simulink model "nfo"  (R2023b)
settings: Solver=FixedStepAuto  StartTime=0.0  StopTime=10.0  FixedStep=1e-4  RelTol=1e-3
values from neighbouring files (symbols this model uses):
  flux = 0.0059    [nfo.sldd]
  if_init = 40.0    [nfo.sldd]
  L = 8.5E-5    [nfo.sldd]
  Pn = 5.0    [nfo.sldd]
  Rs = 0.035    [nfo.sldd]
  Ts = 0.0001    [nfo.sldd]
  Udc = 24.0    [nfo.sldd]
undefined symbols (not defined in the file or in its folder): DiscIntNeverNeededParam, magnitude, PLL_I, PLL_P, sigbuilder_block
libraries: slpidlib x4, dspstat3 x1, mcbplantlib x1, autolibpmsmexterior x1
(part 2 of 2)

== matlab function nfo/Algorithm/Enabled Subsystem/MATLAB Function ==
  data: Time input; Iq output; IF_iq input; Speed_iq input; Cos_eror input; Switch_time input
function Iq = fcn(Time,IF_iq,Speed_iq,Cos_eror,Switch_time)

Iq = IF_iq;

persistent real_iq last_iq
if isempty(real_iq)
    real_iq = Cos_eror;
    last_iq = Iq;
end

if(Time<Switch_time)
    Iq = IF_iq;
    real_iq = Cos_eror;
elseif(Switch_time<=Time && Time<=Switch_time+0.05)
    Iq = 0.059411936635658*real_iq + 0.940588063364342*last_iq; %  0.01/6.125Tc
else
    Iq = Speed_iq;
end

last_iq = Iq;

== stateflow chart nfo/Algorithm/Chart ==
  state out = low_vbus(Input) [function]
  state out = over_vbus(Input) [function]
  state None
    during:
    low = low_vbus(udc);
    over=over_vbus(udc);
    stop = low+over;
    exit:
    low = low_vbus(udc);
    over=over_vbus(udc);
    stop = low+over;
  state Out
    during:
    low=low_vbus(udc);
    over=over_vbus(udc);
    stop=low+over;
    go=1;
  (default) -> None : {udc_max=28;udc_min=15;}
  None -> Out : [run_flag==1 && stop==0]
  Out -> None [order 2] : [run_flag==0]
  Out -> None [order 1] : [over==1 || low==1 || run_flag==0]{go=0}
  data: Input function_input single size=1; out function_output; Input function_input single size=1; out function_output; run_flag input; udc input; udc_max local; udc_min local; low output single; over output single; stop output single =0; go output single =0
